simulink model "home_model"  (R2023b)
settings: Solver=VariableStepAuto  StartTime=0.0  StopTime=43200  MaxStep=0.05  RelTol=1e-3
libraries: SimscapeFluids_lib x32, fl_lib x31, nesl_utility x21
(part 2 of 2)

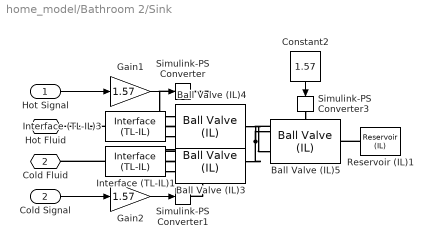
== system home_model/Bathroom 2/Sink ==
  Hot Signal : Inport
  Cold Signal : Inport  Port=2
  Ball Valve (IL)3 : SimscapeFluids_lib/Isothermal Liquid/Valves & Orifices/Flow Control Valves/Ball Valve (IL)  valve_type=fluids.isothermal_liquid.valves_orifices.flow_control_valves.enum.BallValveSpec.Standard  parameterization=fluids.isothermal_liquid.valves_orifices.flow_control_valves.enum.FlowCoefficientSpec.Kv  Cv_max=32 gpm  Kv_max=2 gpm  Cd=0.64  area_port=pi * (75 ^ 2) / 4 mm^2  area_ball=pi * (75 ^ 2) / 4 mm^2  Cv_TLU=[1e-06, .58, 1.15, 1.9, 2.8, 4.3, 7, 10.5, 17, 26, 32] gpm  Kv_TLU=[1e-06, .34, .76, 1.6, 2.45, 4.1, 5.75, 9.4, 13, 28, 50] m^3/hr  area_TLU=[1e-10, 62.5, 125, 187.5, 250, 312.5, 375, 437.5, 500, 562.5, 625] mm^2  rotation_TLU=pi / 2 .* [0, .1, .2, .3, .4, .5, .6, .7, .8, .9, 1] rad  area_leak=1e-10 m^2  Re_c=150  rho_water60F=0.99897 g/cm^3  rho_water15C=0.99913 g/cm^3
      settings: InternalSimscapePortConfiguration="{\"Bottom\":[],\"Left\":[{\"id\":\"A\",\"label\":\"A\",\"type\":\"foundation.isothermal_liquid.isothermal_liquid\"}],\"Right\":[{\"id\":\"B\",\"label\":\"B\",\"type\":\"foundation.isothermal_liquid.isothermal_liquid\"}],\"Top\":[{\"id\":\"S\",\"label\":\"S\",\"type\":\"input\"}]}"
  Ball Valve (IL)4 : SimscapeFluids_lib/Isothermal Liquid/Valves & Orifices/Flow Control Valves/Ball Valve (IL)  valve_type=fluids.isothermal_liquid.valves_orifices.flow_control_valves.enum.BallValveSpec.Standard  parameterization=fluids.isothermal_liquid.valves_orifices.flow_control_valves.enum.FlowCoefficientSpec.Kv  Cv_max=32 gpm  Kv_max=2 gpm  Cd=0.64  area_port=pi * (75 ^ 2) / 4 mm^2  area_ball=pi * (75 ^ 2) / 4 mm^2  Cv_TLU=[1e-06, .58, 1.15, 1.9, 2.8, 4.3, 7, 10.5, 17, 26, 32] gpm  Kv_TLU=[1e-06, .34, .76, 1.6, 2.45, 4.1, 5.75, 9.4, 13, 28, 50] m^3/hr  area_TLU=[1e-10, 62.5, 125, 187.5, 250, 312.5, 375, 437.5, 500, 562.5, 625] mm^2  rotation_TLU=pi / 2 .* [0, .1, .2, .3, .4, .5, .6, .7, .8, .9, 1] rad  area_leak=1e-10 m^2  Re_c=150  rho_water60F=0.99897 g/cm^3  rho_water15C=0.99913 g/cm^3
      settings: InternalSimscapePortConfiguration="{\"Bottom\":[],\"Left\":[{\"id\":\"A\",\"label\":\"A\",\"type\":\"foundation.isothermal_liquid.isothermal_liquid\"}],\"Right\":[{\"id\":\"B\",\"label\":\"B\",\"type\":\"foundation.isothermal_liquid.isothermal_liquid\"}],\"Top\":[{\"id\":\"S\",\"label\":\"S\",\"type\":\"input\"}]}"
  Ball Valve (IL)5 : SimscapeFluids_lib/Isothermal Liquid/Valves & Orifices/Flow Control Valves/Ball Valve (IL)  valve_type=fluids.isothermal_liquid.valves_orifices.flow_control_valves.enum.BallValveSpec.Standard  parameterization=fluids.isothermal_liquid.valves_orifices.flow_control_valves.enum.FlowCoefficientSpec.Kv  Cv_max=32 gpm  Kv_max=2 gpm  Cd=0.64  area_port=pi * (25 ^ 2) / 4 mm^2  area_ball=pi * (20 ^ 2) / 4 mm^2  Cv_TLU=[1e-06, .58, 1.15, 1.9, 2.8, 4.3, 7, 10.5, 17, 26, 32] gpm  Kv_TLU=[1e-06, .34, .76, 1.6, 2.45, 4.1, 5.75, 9.4, 13, 28, 50] m^3/hr  area_TLU=[1e-10, 62.5, 125, 187.5, 250, 312.5, 375, 437.5, 500, 562.5, 625] mm^2  rotation_TLU=pi / 2 .* [0, .1, .2, .3, .4, .5, .6, .7, .8, .9, 1] rad  area_leak=1e-10 m^2  Re_c=150  rho_water60F=0.99897 g/cm^3  rho_water15C=0.99913 g/cm^3
      settings: InternalSimscapePortConfiguration="{\"Bottom\":[],\"Left\":[{\"id\":\"A\",\"label\":\"A\",\"type\":\"foundation.isothermal_liquid.isothermal_liquid\"}],\"Right\":[{\"id\":\"B\",\"label\":\"B\",\"type\":\"foundation.isothermal_liquid.isothermal_liquid\"}],\"Top\":[{\"id\":\"S\",\"label\":\"S\",\"type\":\"input\"}]}"
  Constant2 : Constant  Value=1.57
  Gain1 : Gain  Gain=1.57
  Gain2 : Gain  Gain=1.57
  Interface (TL-IL)1 : SimscapeFluids_lib/Fluid Network Interfaces/Interface (TL-IL)  interface_domain_spec=fluids.interfaces.enum.interface_domain_spec.TL_IL  temperature_spec=foundation.enum.constant_controlled.constant  T_interface=293.15 K  area_TL=0.01 m^2
      settings: InternalSimscapePortConfiguration="{\"Bottom\":[],\"Left\":[{\"id\":\"TL\",\"label\":\"TL\",\"type\":\"foundation.thermal_liquid.thermal_liquid\"}],\"Right\":[{\"id\":\"IL\",\"label\":\"IL\",\"type\":\"foundation.isothermal_liquid.isothermal_liquid\"}],\"Top\":[]}"
  Interface (TL-IL)3 : SimscapeFluids_lib/Fluid Network Interfaces/Interface (TL-IL)  interface_domain_spec=fluids.interfaces.enum.interface_domain_spec.TL_IL  temperature_spec=foundation.enum.constant_controlled.constant  T_interface=293.15 K  area_TL=0.01 m^2
      settings: InternalSimscapePortConfiguration="{\"Bottom\":[],\"Left\":[{\"id\":\"TL\",\"label\":\"TL\",\"type\":\"foundation.thermal_liquid.thermal_liquid\"}],\"Right\":[{\"id\":\"IL\",\"label\":\"IL\",\"type\":\"foundation.isothermal_liquid.isothermal_liquid\"}],\"Top\":[]}"
  Reservoir (IL)1 : fl_lib/Isothermal Liquid/Elements/Reservoir (IL)  reservoir_type=foundation.enum.constant_controlled.constant  pressure_spec=foundation.enum.pressure_spec.atmospheric  reservoir_pressure=0.101325 MPa
  Simulink-PS Converter : nesl_utility/Simulink-PS Converter  PhysicalDomain=network_engine_domain  SubClassName=ps_input  LeftPortType=input  RightPortType=output  PseudoPeriodic=off  Frequencies=[]  NoiseDistribution=none  NoiseParameters=[]  Unit=1  AffineConversion=off  FilteringAndDerivatives=provide  SimscapeFilterOrder=1  InputFilterTimeConstant=0.001  UdotUserProvided=0
  Simulink-PS Converter1 : nesl_utility/Simulink-PS Converter  PhysicalDomain=network_engine_domain  SubClassName=ps_input  LeftPortType=input  RightPortType=output  PseudoPeriodic=off  Frequencies=[]  NoiseDistribution=none  NoiseParameters=[]  Unit=1  AffineConversion=off  FilteringAndDerivatives=provide  SimscapeFilterOrder=1  InputFilterTimeConstant=0.001  UdotUserProvided=0
  Simulink-PS Converter3 : nesl_utility/Simulink-PS Converter  PhysicalDomain=network_engine_domain  SubClassName=ps_input  LeftPortType=input  RightPortType=output  PseudoPeriodic=off  Frequencies=[]  NoiseDistribution=none  NoiseParameters=[]  Unit=1  AffineConversion=off  FilteringAndDerivatives=provide  SimscapeFilterOrder=1  InputFilterTimeConstant=0.001  UdotUserProvided=0
  Hot Fluid : PMIOPort  Side=Left
  Cold Fluid : PMIOPort  Port=2  Side=Left
  wires:
  Constant2/1 -> Simulink-PS Converter3/1
  Hot Signal/1 -> Gain1/1
  Gain1/1 -> Simulink-PS Converter/1
  Gain2/1 -> Simulink-PS Converter1/1
  Cold Signal/1 -> Gain2/1
  connections:
  Ball Valve (IL)3/RConn1 -- Ball Valve (IL)5/LConn1 -- Ball Valve (IL)4/RConn1
  Simulink-PS Converter3/RConn1 -- Ball Valve (IL)5/LConn2
  Reservoir (IL)1/LConn1 -- Ball Valve (IL)5/RConn1
  Interface (TL-IL)3/LConn1 -- Hot Fluid/RConn1
  Interface (TL-IL)3/RConn1 -- Ball Valve (IL)4/LConn1
  Interface (TL-IL)1/LConn1 -- Cold Fluid/RConn1
  Interface (TL-IL)1/RConn1 -- Ball Valve (IL)3/LConn1
  Simulink-PS Converter/RConn1 -- Ball Valve (IL)4/LConn2
  Ball Valve (IL)3/LConn2 -- Simulink-PS Converter1/RConn1

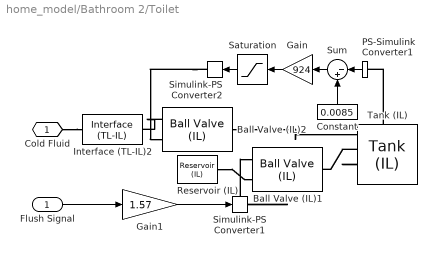
== system home_model/Bathroom 2/Toilet ==
  Flush Signal : Inport
  Ball Valve (IL)1 : SimscapeFluids_lib/Isothermal Liquid/Valves & Orifices/Flow Control Valves/Ball Valve (IL)  valve_type=fluids.isothermal_liquid.valves_orifices.flow_control_valves.enum.BallValveSpec.Standard  parameterization=fluids.isothermal_liquid.valves_orifices.flow_control_valves.enum.FlowCoefficientSpec.Kv  Cv_max=32 gpm  Kv_max=49 m^3/hr  Cd=0.64  area_port=pi * (75 ^ 2) / 4 mm^2  area_ball=pi * (75 ^ 2) / 4 mm^2  Cv_TLU=[1e-06, .58, 1.15, 1.9, 2.8, 4.3, 7, 10.5, 17, 26, 32] gpm  Kv_TLU=[1e-06, .34, .76, 1.6, 2.45, 4.1, 5.75, 9.4, 13, 28, 50] m^3/hr  area_TLU=[1e-10, 62.5, 125, 187.5, 250, 312.5, 375, 437.5, 500, 562.5, 625] mm^2  rotation_TLU=pi / 2 .* [0, .1, .2, .3, .4, .5, .6, .7, .8, .9, 1] rad  area_leak=1e-10 m^2  Re_c=150  rho_water60F=0.99897 g/cm^3  rho_water15C=0.99913 g/cm^3
      settings: InternalSimscapePortConfiguration="{\"Bottom\":[],\"Left\":[{\"id\":\"A\",\"label\":\"A\",\"type\":\"foundation.isothermal_liquid.isothermal_liquid\"}],\"Right\":[{\"id\":\"B\",\"label\":\"B\",\"type\":\"foundation.isothermal_liquid.isothermal_liquid\"}],\"Top\":[{\"id\":\"S\",\"label\":\"S\",\"type\":\"input\"}]}"
  Ball Valve (IL)2 : SimscapeFluids_lib/Isothermal Liquid/Valves & Orifices/Flow Control Valves/Ball Valve (IL)  valve_type=fluids.isothermal_liquid.valves_orifices.flow_control_valves.enum.BallValveSpec.Standard  parameterization=fluids.isothermal_liquid.valves_orifices.flow_control_valves.enum.FlowCoefficientSpec.Kv  Cv_max=32 gpm  Kv_max=2.25 gpm  Cd=0.64  area_port=pi * (9.525 ^ 2) / 4 mm^2  area_ball=pi * (9.525 ^ 2) / 4 mm^2  Cv_TLU=[1e-06, .58, 1.15, 1.9, 2.8, 4.3, 7, 10.5, 17, 26, 32] gpm  Kv_TLU=[1e-06, .34, .76, 1.6, 2.45, 4.1, 5.75, 9.4, 13, 28, 50] m^3/hr  area_TLU=[1e-10, 62.5, 125, 187.5, 250, 312.5, 375, 437.5, 500, 562.5, 625] mm^2  rotation_TLU=pi / 2 .* [0, .1, .2, .3, .4, .5, .6, .7, .8, .9, 1] rad  area_leak=1e-10 m^2  Re_c=150  rho_water60F=0.99897 g/cm^3  rho_water15C=0.99913 g/cm^3
      settings: InternalSimscapePortConfiguration="{\"Bottom\":[],\"Left\":[{\"id\":\"A\",\"label\":\"A\",\"type\":\"foundation.isothermal_liquid.isothermal_liquid\"}],\"Right\":[{\"id\":\"B\",\"label\":\"B\",\"type\":\"foundation.isothermal_liquid.isothermal_liquid\"}],\"Top\":[{\"id\":\"S\",\"label\":\"S\",\"type\":\"input\"}]}"
  Constant : Constant  Value=0.0085
  Gain : Gain  Gain=924
  Gain1 : Gain  Gain=1.57
  Interface (TL-IL)2 : SimscapeFluids_lib/Fluid Network Interfaces/Interface (TL-IL)  interface_domain_spec=fluids.interfaces.enum.interface_domain_spec.TL_IL  temperature_spec=foundation.enum.constant_controlled.constant  T_interface=293.15 K  area_TL=0.01 m^2
      settings: InternalSimscapePortConfiguration="{\"Bottom\":[],\"Left\":[{\"id\":\"TL\",\"label\":\"TL\",\"type\":\"foundation.thermal_liquid.thermal_liquid\"}],\"Right\":[{\"id\":\"IL\",\"label\":\"IL\",\"type\":\"foundation.isothermal_liquid.isothermal_liquid\"}],\"Top\":[]}"
  PS-Simulink Converter1 : nesl_utility/PS-Simulink Converter  PhysicalDomain=network_engine_domain  SubClassName=ps_output  LeftPortType=input  RightPortType=output  PseudoPeriodic=off  Frequencies=[]  VectorFormat=inherit  Unit=inherit  AffineConversion=off
  Reservoir (IL) : fl_lib/Isothermal Liquid/Elements/Reservoir (IL)  reservoir_type=foundation.enum.constant_controlled.constant  pressure_spec=foundation.enum.pressure_spec.atmospheric  reservoir_pressure=0.101325 MPa
  Saturation : Saturate  UpperLimit=1.5707  LowerLimit=0
  Simulink-PS Converter1 : nesl_utility/Simulink-PS Converter  PhysicalDomain=network_engine_domain  SubClassName=ps_input  LeftPortType=input  RightPortType=output  PseudoPeriodic=off  Frequencies=[]  NoiseDistribution=none  NoiseParameters=[]  Unit=1  AffineConversion=off  FilteringAndDerivatives=provide  SimscapeFilterOrder=1  InputFilterTimeConstant=0.001  UdotUserProvided=0
  Simulink-PS Converter2 : nesl_utility/Simulink-PS Converter  PhysicalDomain=network_engine_domain  SubClassName=ps_input  LeftPortType=input  RightPortType=output  PseudoPeriodic=off  Frequencies=[]  NoiseDistribution=none  NoiseParameters=[]  Unit=1  AffineConversion=off  FilteringAndDerivatives=provide  SimscapeFilterOrder=1  InputFilterTimeConstant=0.001  UdotUserProvided=0
  Sum : Sum  Inputs=|-+
  Tank (IL) : SimscapeFluids_lib/Isothermal Liquid/Tanks & Accumulators/Tank (IL)  num_inlet=fluids.isothermal_liquid.tanks_accumulators.enum.NumInlet.Two  pressure_spec=fluids.isothermal_liquid.tanks_accumulators.enum.TankPressureSpec.Atmospheric  tank_pressure=0.101325 MPa  volume_spec=fluids.isothermal_liquid.tanks_accumulators.enum.TankVolumeSpec.Constant  tank_area=0.135 m^2  level_TLU=[0, 3, 5] m  volume_TLU=[0, 4, 6] m^3  inlet_height_A=0.1 m  inlet_area_A=0.01 m^2  inlet_height_AB=[0,0] m  inlet_area_AB=[.442,7] in^2  inlet_height_ABC=[.1, .1, .1] m  inlet_area_ABC=[.01, .01, .01] m^2  inlet_height_ABCD=0.1 * ones(1, 4) m  inlet_area_ABCD=0.01 * ones(1, 4) m^2  inlet_height_ABCDE=0.1 * ones(1, 5) m  inlet_area_ABCDE=0.01 * ones(1, 5) m^2  inlet_height_ABCDEF=0.1 * ones(1, 6) m  inlet_area_ABCDEF=0.01 * ones(1, 6) m^2  level_check=simscape.enum.assert.action.none  capacity_check=simscape.enum.assert.action.none  max_capacity=10 m^3  g=9.81 m/s^2  level_specify=off  level_priority=High  level=5 m  level_nominal_specify=off  level_nominal_unit=m  level_nominal_value=1  volume_specify=on  volume_priority=High  volume=2 gal  volume_nominal_specify=off  volume_nominal_unit=m^3  volume_nominal_value=1  mass_specify=off  mass_priority=None  mass=5000 kg  mass_nominal_specify=off  mass_nominal_unit=kg  mass_nominal_value=1
      settings: InternalSimscapePortConfiguration="{\"Bottom\":[],\"Left\":[{\"id\":\"A\",\"label\":\"A\",\"type\":\"foundation.isothermal_liquid.isothermal_liquid\"},{\"id\":\"B\",\"label\":\"B\",\"type\":\"foundation.isothermal_liquid.isothermal_liquid\"}],\"Right\":[],\"Top\":[{\"id\":\"V\",\"label\":\"V\",\"type\":\"output\"},{\"id\":\"L\",\"label\":\"L\",\"type\":\"output\"}]}"
  Cold Fluid : PMIOPort  Side=Left
  wires:
  Flush Signal/1 -> Gain1/1
  Gain1/1 -> Simulink-PS Converter1/1
  PS-Simulink Converter1/1 -> Sum/1
  Sum/1 -> Gain/1
  Constant/1 -> Sum/2
  Saturation/1 -> Simulink-PS Converter2/1
  Gain/1 -> Saturation/1
  connections:
  Simulink-PS Converter2/RConn1 -- Ball Valve (IL)2/LConn2
  Ball Valve (IL)2/LConn1 -- Interface (TL-IL)2/RConn1
  Tank (IL)/LConn3 -- PS-Simulink Converter1/LConn1
  Ball Valve (IL)2/RConn1 -- Tank (IL)/LConn1
  Tank (IL)/LConn2 -- Ball Valve (IL)1/RConn1
  Simulink-PS Converter1/RConn1 -- Ball Valve (IL)1/LConn2
  Reservoir (IL)/LConn1 -- Ball Valve (IL)1/LConn1
  Cold Fluid/RConn1 -- Interface (TL-IL)2/LConn1
